simulink model "FullHopper_passiveExo_PWM"  (R2020b)
settings: Solver=ode4  StartTime=0  StopTime=20  FixedStep=0.0005  RelTol=1e-7  AbsTol=1e-9  EnableMultiTasking=on
settings Model: Creator=Laksh  LastModifiedBy=ishratarora
settings SolverCC: AutoScaleAbsTol=off  MaxConsecutiveMinStep=10  AlgebraicLoopSolver=LineSearch
settings DataIOCC: SaveFormat=StructureWithTime  SignalLogging=off
settings OptimizationCC: LifeSpan=inf
settings DebuggingCC: ReadBeforeWriteMsg=DisableAll  WriteAfterWriteMsg=DisableAll  WriteAfterReadMsg=DisableAll  AlgebraicLoopMsg=none  MultiTaskDSMMsg=none  SFUnexpectedBacktrackingDiag=warning  SFNoUnconditionalDefaultTransitionDiag=warning  SFExecutionAtInitializationDiag=none  ArithmeticOperatorsInVariantConditions=warning
settings ModelReferenceCC: UpdateModelReferenceTargets=IfOutOfDate  ModelReferenceMinAlgLoopOccurrences=on
settings SFSimCC: SFSimEcho=off  SimUseLocalCustomCode=off  CustomCodeUndefinedFunction=UseInterfaceOnly
settings RTWCC: RTWUseLocalCustomCode=off
settings CodeAppCC: StateflowObjectComments=on
settings GRTTargetCC: TargetLangStandard=C89/C90 (ANSI)
settings ConfigComp: CovMetricSettings=dw  CovSaveCumulativeToWorkspaceVar=on  CovSaveSingleToWorkspaceVar=on  CovExternalEMLEnable=off

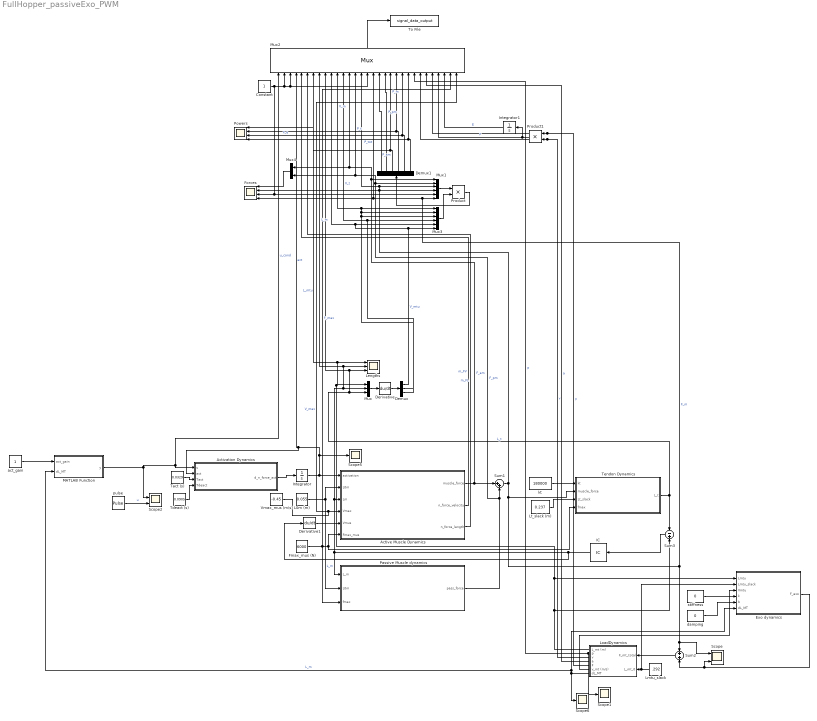
== system FullHopper_passiveExo_PWM ==
  Activation Dynamics : MATLAB Function  TreatAsAtomicUnit=on
  Active Muscle Dynamics : MATLAB Function
  Constant : Constant
  Demux : Demux  Outputs=3
  Demux1 : Demux  Outputs=6
  Derivative : Derivative
  Derivative1 : Derivative
  Exo dynamics : MATLAB Function  TreatAsAtomicUnit=on
  Fmax_mus (N) : Constant  Value=6000
  Forces : Scope  NumInputPorts=4
  IC : InitialCondition  Value=0.055
  Integrator : Integrator
  Integrator1 : Integrator
  L0m (m) : Constant  Value=0.055
  Lengths : Scope  NumInputPorts=3
  Lmtu_slack : Constant  Value=.292
  LoadDynamics : Subsystem
  Lt_slack (m) : Constant  Value=0.237
  MATLAB Function : MATLAB Function  TreatAsAtomicUnit=on
  Mux : Mux  Inputs=3
  Mux1 : Mux  Inputs=6
  Mux2 : Mux  Inputs=31
      settings: DisplayOption=signals
  Mux3 : Mux  Inputs=6
  Mux4 : Mux  Inputs=2
  Passive Muscle dynamics : MATLAB Function
  Powers : Scope  NumInputPorts=4
  Product : Product
  Product1 : Product
  Scope : Scope  NumInputPorts=2
  Scope1 : Scope
  Scope2 : Scope  NumInputPorts=2
  Scope5 : Scope
  Scope6 : Scope
  Sum1 : Sum  Inputs=|++
  Sum2 : Sum  Inputs=+|+
  Sum3 : Sum  Inputs=-|+
  Tact (s) : Constant  Value=0.0329  VectorParams1D=off
  Tdeact (s) : Constant  Value=0.0905
  Tendon Dynamics : MATLAB Function
  To File : ToFile  Filename=signal_data_output  MatrixName=data  SaveFormat=Timeseries
  Vmax_mus (m\s) : Constant  Value=-0.45
  act_gain : Constant
  damping : Constant  Value=0
  kt : Constant  Value=180000
  pulse : DiscretePulseGenerator  PulseType=Time based  Period=0.4  PulseWidth=10
  stiffness : Constant  Value=0
  wires:
  Activation Dynamics/1(d_n_force_act) -> Integrator/1
  Integrator/1 -> Scope5/1, Activation Dynamics/2(act), Mux2/4, Active Muscle Dynamics/1(activation)  "act"
  Tact (s)/1 -> Activation Dynamics/3(Tact)
  Tdeact (s)/1 -> Activation Dynamics/4(Tdeact)
  L0m (m)/1 -> Active Muscle Dynamics/2(L0m), Passive Muscle dynamics/2(L0m)  "L_m"
  Vmax_mus (m\s)/1 -> Mux2/31, Active Muscle Dynamics/4(Vmax)  "V_max"
  Passive Muscle dynamics/1(pass_force) -> Mux1/2, Mux4/2, Mux2/14, Sum1/2  "F_pm"
  Sum1/1 -> Mux1/4, Mux1/3, Mux2/15, Forces/2, Scope/1, Sum2/1, Mux1/6, Forces/4, Mux2/17, Tendon Dynamics/2(muscle_force)  "F_m"
  Lt_slack (m)/1 -> Tendon Dynamics/3(Lt_slack)
  kt/1 -> Tendon Dynamics/1(kt)
  LoadDynamics/1(L_mt (m)) -> Sum3/2, Lengths/1, Mux2/7, Mux/1, Exo dynamics/1(Lmtu)  "L_mtu"
  Active Muscle Dynamics/1(muscle_force) -> Sum1/1, Mux1/1, Mux4/1, Mux2/13  "F_am"
  Mux2/1 -> To File/1
  Lmtu_slack/1 -> Exo dynamics/2(Lmtu_slack), LoadDynamics/2(L_mt_0)
  Active Muscle Dynamics/2(n_force_velocity) -> Mux2/5  "m_FV"
  Active Muscle Dynamics/3(n_force_length) -> Mux2/6  "m_FL"
  Mux/1 -> Derivative/1
  Derivative/1 -> Demux/1
  Demux/1 -> Mux3/5, Mux2/10, Mux3/6  "V_mtu"
  Demux/2 -> Mux3/3, Mux3/2, Mux3/1, Mux2/11  "V_m"
  Demux/3 -> Mux3/4, Mux2/12  "V_t"
  Mux1/1 -> Product/1
  Mux3/1 -> Product/2
  Product/1 -> Demux1/1
  Demux1/1 -> Mux2/18  "P_am"
  Demux1/2 -> Mux2/19  "P_pm"
  Demux1/3 -> Mux2/20, Powers/1  "P_m"
  Demux1/4 -> Mux2/21, Powers/2  "P_t"
  Demux1/5 -> Mux2/22, Powers/3  "P_e"
  Demux1/6 -> Mux2/23, Powers/4  "P_tot"
  LoadDynamics/2(p) -> Scope1/1, Mux2/24  "p"
  LoadDynamics/3(v) -> Mux2/25, Product1/2  "v"
  LoadDynamics/4(a) -> Mux2/26  "a"
  LoadDynamics/5(F) -> Mux2/27, Product1/1  "F"
  Product1/1 -> Mux2/28, Integrator1/1  "P"
  Integrator1/1 -> Mux2/29  "E"
  Tendon Dynamics/1(L_t) -> Lengths/3, Mux2/9, Mux/3, Sum3/1  "L_t"
  Sum3/1 -> IC/1
  IC/1 -> Derivative1/1, Passive Muscle dynamics/1(L_m), Mux/2, Lengths/2, Mux2/8, Active Muscle Dynamics/3(Lm)  "L_m"
  Derivative1/1 -> Active Muscle Dynamics/5(Vmus)
  Mux4/1 -> Forces/1
  MATLAB Function/1(y) -> Mux2/1, Activation Dynamics/1(u), Scope2/1  "u_cond"
  LoadDynamics/6(v_mt (m/s)) -> Exo dynamics/3(Vmtu)
  Constant/1 -> Mux1/5, Forces/3, Mux2/16, Mux2/3, Mux2/2
  damping/1 -> Exo dynamics/5(b)
  stiffness/1 -> Exo dynamics/4(k)
  Sum2/1 -> LoadDynamics/1(F_mt_total)
  Exo dynamics/1(F_exo) -> Sum2/2, Scope/2
  pulse/1 -> Scope2/2  "u"
  Fmax_mus (N)/1 -> Active Muscle Dynamics/6(Fmax_mus), Tendon Dynamics/4(fmax), Mux2/30, Passive Muscle dynamics/3(fmax)  "F_max"
  LoadDynamics/7(dL_MT) -> MATLAB Function/2(dL_MT), Exo dynamics/6(dL_MT), Scope6/1  "L_m"
  act_gain/1 -> MATLAB Function/1(act_gain)

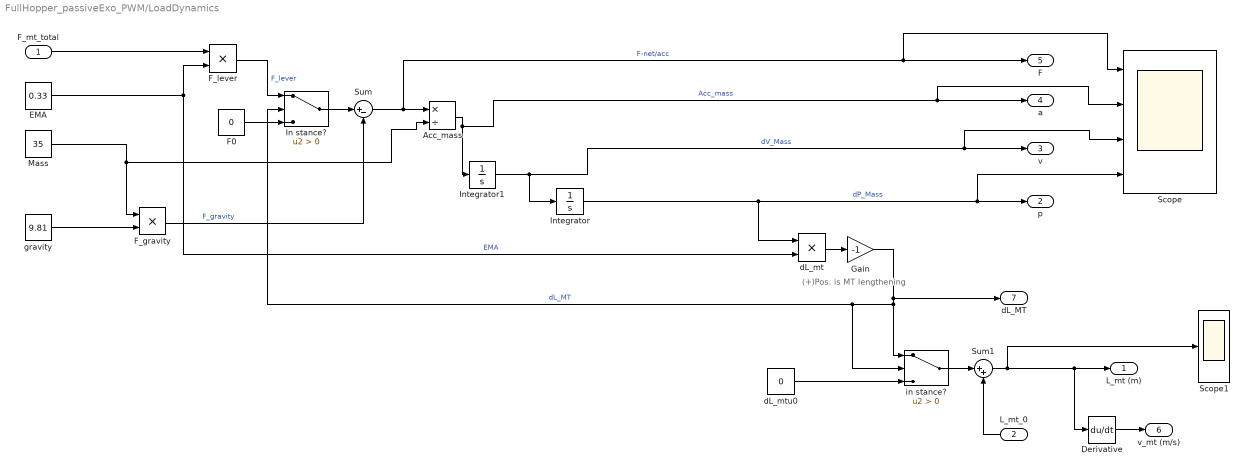
== system FullHopper_passiveExo_PWM/LoadDynamics ==
  note: (+)Pos. is MT
      | lengthening
  F_mt_total : Inport
  L_mt_0 : Inport  Port=2
  Acc_mass : Product  Inputs=*/
  Derivative : Derivative
  EMA : Constant  Value=0.33
  F0 : Constant  Value=0
  F_gravity : Product  RndMeth=Zero
  F_lever : Product  RndMeth=Zero
  Gain : Gain  Gain=-1
  In stance? : Switch  Criteria=u2 > Threshold
  Integrator : Integrator  InitialCondition=0.1
  Integrator1 : Integrator
  Mass : Constant  Value=35
  Scope : Scope  NumInputPorts=4
  Scope1 : Scope
  Sum : Sum  Inputs=|+-
  Sum1 : Sum  Inputs=|++
  dL_mt : Product  RndMeth=Zero
  dL_mtu0 : Constant  Value=0
  gravity : Constant  Value=9.81
  "in stance? " : Switch  Criteria=u2 > Threshold
  L_mt (m) : Outport
  p : Outport  Port=2
  v : Outport  Port=3
  a : Outport  Port=4
  F : Outport  Port=5
  v_mt (m/s) : Outport  Port=6
  dL_MT : Outport  Port=7
  wires:
  Integrator1/1 -> Integrator/1, Scope/3, v/1  "dV_Mass"
  Sum1/1 -> Scope1/1, Derivative/1, L_mt (m)/1
  L_mt_0/1 -> Sum1/2
  Acc_mass/1 -> Integrator1/1, Scope/2, a/1  "Acc_mass"
  F0/1 -> In stance?/3
  Sum/1 -> Scope/1, F/1, Acc_mass/1  "F-net/acc"
  F_mt_total/1 -> F_lever/1
  Gain/1 -> "in stance? "/1, "in stance? "/2, In stance?/2, dL_MT/1  "dL_MT"
  dL_mt/1 -> Gain/1
  F_lever/1 -> In stance?/1  "F_lever"
  Integrator/1 -> dL_mt/1, Scope/4, p/1  "dP_Mass"
  F_gravity/1 -> Sum/2  "F_gravity"
  EMA/1 -> F_lever/2, dL_mt/2  "EMA"
  gravity/1 -> F_gravity/2
  Mass/1 -> Acc_mass/2, F_gravity/1
  dL_mtu0/1 -> "in stance? "/3
  In stance?/1 -> Sum/1
  "in stance? "/1 -> Sum1/1
  Derivative/1 -> v_mt (m/s)/1

== matlab function FullHopper_passiveExo_PWM/Exo dynamics ==
  data: Lmtu input; Lmtu_slack input; F_exo output; Vmtu input; k input; b input; dL_MT input
function F_exo  = exo_dynamics(Lmtu, Lmtu_slack, Vmtu, k, b, dL_MT)

dL_MT = -dL_MT;

    if dL_MT > 0 %Check if landing
        F_exo = k*(Lmtu-Lmtu_slack) - Vmtu*b;

    else 
        F_exo = k*(Lmtu-Lmtu_slack);
    end

end

== matlab function FullHopper_passiveExo_PWM/Active Muscle Dynamics ==
  data: activation input; L0m input; Lm input; Vmax input; Vmus input; Fmax_mus input; muscle_force output; n_force_velocity output; n_force_length output
function [muscle_force, n_force_velocity, n_force_length]  =...
    muscle_dynamics(activation,L0m,Lm,Vmax,Vmus,Fmax_mus)
%#codegen

    %Hill Type Muscle F-V relationship.  Returns a normalized force-velocity value
    if (Vmus<Vmax)
        n_force_velocity=0;
    else
        if (Vmus >= Vmax && Vmus < 0)
            n_force_velocity = ((1-(Vmus/Vmax))/(1+(Vmus/0.17/Vmax)));
        else
            n_force_velocity =(1.8-0.8*((1+(Vmus/Vmax))/(1-7.56*Vmus/0.17/Vmax)));
        end
    end
    
    %Active muscle F-L relationships.  Returns a normalized F-L value

    a = 3.1108;
    b = .8698;
    s = .3914;

    if Lm < 0
        Lm = 0;
    end

    n_force_length = exp(-(abs(((Lm/L0m)^b-1)/s))^a);

    %Total active force of muscle based on normalized F-V and F-L relationships
    muscle_force = Fmax_mus* activation * n_force_velocity * n_force_length;
end

== matlab function FullHopper_passiveExo_PWM/Tendon Dynamics ==
  data: kt input; L_t output; muscle_force input; Lt_slack input; fmax input
function L_t = L_tendon(kt,muscle_force,Lt_slack,fmax)
%#codegen

%Total tendon length
%kt_comp = @(fm) 1./(kt*(1+(0.9./((-exp((20*fm)./fmax))))));
dL_t = ((muscle_force + (fmax*log((-9*exp(-(20*muscle_force)/fmax)) + 10))/20)/kt);
L_t = dL_t + Lt_slack ;

end

== matlab function FullHopper_passiveExo_PWM/Activation Dynamics ==
  data: u input; d_n_force_act output; act input; Tact input; Tdeact input
function d_n_force_act = d_n_force_act(u,act,Tact,Tdeact)
%#codegen    
%Rate of change of activation
    B=Tact/Tdeact;
    d_n_force_act= u/Tact - (1/Tact*(B+(1-B)*u))*act;
end

== matlab function FullHopper_passiveExo_PWM/Passive Muscle dynamics ==
  data: pass_force output; L_m input; L0m input; fmax input
function pass_force = pmuscle_dynamics(L_m, L0m,fmax)
%#codegen
%passive CE F_L taken from Rubenson et. al.

%Passive muscle force
A = 2.38*10^(-2);
b = 5.31;

if L_m > 0    
    pass_force= fmax*A*exp(b*((L_m/L0m)-1));
else
    pass_force=0;
end


end

== matlab function FullHopper_passiveExo_PWM/MATLAB Function ==
  settings: updateMethod=DISCRETE
  data: act_gain input; dL_MT input; y output
function y = PWM_trigger(act_gain, dL_MT)

persistent tick vec started


if isempty(tick)
    tick = 0;
    vec = 0;
    started = 0;
end

y = 0;

%Check sign of dL_MT
if dL_MT > 0
    value = 1; 
else 
    value = 0;
end

vec = [vec value];

%Check currently positive and previously negative
if vec(end) && ~vec(end-1)
    started = 1;
end

if started
    if tick<80
        tick=tick+1;
        y = 1 * act_gain;
    else
        tick = 0;
        started = 0;
    end 
end



end
